simulink model "controller_v11_run"  (R2023a)
settings: Solver=ode4  StartTime=0.0  StopTime=5  FixedStep=0.00001  RelTol=1e-3
values from neighbouring files (symbols this model uses):
  m = 6    [coordinator_v2.m]
  N = 10    [coordinator_v2.m]
undefined symbols (not defined in the file or in its folder): PD_result, sd, X, Y, Z
libraries: sm_lib x191, nesl_utility x71
(part 1 of 5)
settings Model: Creator=25394  LastModifiedBy=shiyi
settings OptimizationCC: ReuseModelBlockBuffer=off

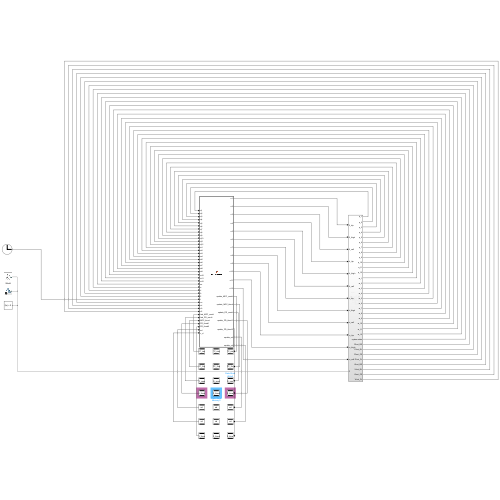
[thumbnail: Simulink's stored preview of the top-level diagram]
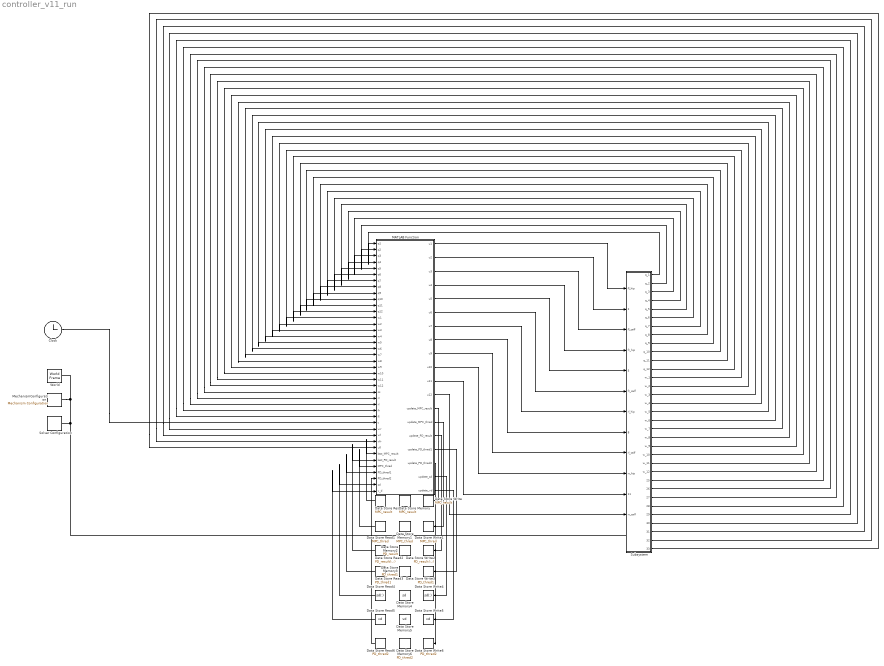
== system controller_v11_run ==
  Clock : Clock
  Data Store Memory : DataStoreMemory  DataStoreName=MPC_result  WriteAfterWriteMsg=warning  InitialValue=[0; 0; 0; 0; 0; 0; 0; 0; 0; 0; 0; 0]  ShowAdditionalParam=off
  Data Store Memory1 : DataStoreMemory  DataStoreName=MPC_thred  WriteAfterWriteMsg=warning  ShowAdditionalParam=off
  Data Store Memory2 : DataStoreMemory  DataStoreName=PD_result  WriteAfterWriteMsg=warning  InitialValue=zeros(24,14)  ShowAdditionalParam=off
  Data Store Memory3 : DataStoreMemory  DataStoreName=PD_thred1  WriteAfterWriteMsg=warning  ShowAdditionalParam=off
  Data Store Memory4 : DataStoreMemory  DataStoreName=sd  WriteAfterWriteMsg=warning  InitialValue=[0.1902; 0; 0.29; 0; 0; 0; 0; 0; 0; 0; 0; 0; 9.81]  ShowAdditionalParam=off
  Data Store Memory5 : DataStoreMemory  DataStoreName=vd  WriteAfterWriteMsg=warning  ShowAdditionalParam=off
  Data Store Memory6 : DataStoreMemory  DataStoreName=PD_thred2  WriteAfterWriteMsg=warning  ShowAdditionalParam=off
  Data Store Read : DataStoreRead  DataStoreName=MPC_result  IndexOptions=Index vector (dialog)  Indices=1  OutputSizes=1
  Data Store Read1 : DataStoreRead  DataStoreName=MPC_thred  IndexOptions=Index vector (dialog)  Indices=1  OutputSizes=1
  Data Store Read2 : DataStoreRead  DataStoreName=PD_result  DataStoreElements=PD_result(:,:)  IndexOptions=Index vector (dialog)  Indices=1  OutputSizes=1
  Data Store Read3 : DataStoreRead  DataStoreName=PD_thred1  IndexOptions=Index vector (dialog)  Indices=1  OutputSizes=1
  Data Store Read4 : DataStoreRead  DataStoreName=sd  DataStoreElements=sd(:)  IndexOptions=Index vector (dialog)  Indices=1  OutputSizes=1
  Data Store Read5 : DataStoreRead  DataStoreName=vd  DataStoreElements=vd  IndexOptions=Index vector (dialog)  Indices=1  OutputSizes=1
  Data Store Read6 : DataStoreRead  DataStoreName=PD_thred2  IndexOptions=Index vector (dialog)  Indices=1  OutputSizes=1
  Data Store Write : DataStoreWrite  DataStoreName=MPC_result  IndexOptions=Index vector (dialog)  Indices=1  OutputSizes=1
  Data Store Write1 : DataStoreWrite  DataStoreName=MPC_thred  IndexOptions=Index vector (dialog)  Indices=1  OutputSizes=1
  Data Store Write2 : DataStoreWrite  DataStoreName=PD_result  DataStoreElements=PD_result(:,:)  IndexOptions=Index vector (dialog)  Indices=1  OutputSizes=1
  Data Store Write3 : DataStoreWrite  DataStoreName=PD_thred1  IndexOptions=Index vector (dialog)  Indices=1  OutputSizes=1
  Data Store Write4 : DataStoreWrite  DataStoreName=sd  DataStoreElements=sd(:)  IndexOptions=Index vector (dialog)  Indices=1  OutputSizes=1
  Data Store Write5 : DataStoreWrite  DataStoreName=vd  DataStoreElements=vd  IndexOptions=Index vector (dialog)  Indices=1  OutputSizes=1
  Data Store Write6 : DataStoreWrite  DataStoreName=PD_thred2  IndexOptions=Index vector (dialog)  Indices=1  OutputSizes=1
  MATLAB Function : MATLAB Function  TreatAsAtomicUnit=on
  MechanismConfiguration : sm_lib/Utilities/Mechanism Configuration  UniformGravity=Constant  GravityVector=[0 0 -9.80665]  GravityVectorUnits=m/s^2  LinearizationDelta=0.001  JointModeTransitionNonlinearIterations=2
  Solver Configuration : nesl_utility/Solver Configuration  PhysicalDomain=network_engine_domain  SubClassName=solver  LeftPortType=input  RightPortType=generic  Tones=[]  Harmonics=[]  SimulateNoise=off  Profile=off  UseLocalSampling=off  EnableSwitchedLinearOptims=on  FrequencyDomain=off  UseCCode=off  RelTol=0.001  AbsTol=0.001  MinStep=1e-09  ToWorkspace=off  RevertToSquareIcSolve=off  NumHomotopyIterations=100  PhasorMode=off  PhasorModeNumHarmonics=1  ConsistencySolver=NEWTON_XTOL_AFTER_FTOL  IndexReductionMethod=DerivativeReplacement  DoDC=off  ResidualTolerance=1e-09  ConsistencyTolSource=GLOBAL  ConsistencyAbsTol=0.001  ConsistencyRelTol=0.001  ConsistencyTolFactor=0.001  UseLocalSolver=off  LocalSolverChoice=NE_BACKWARD_EULER_ADVANCER  ResolveIndetEquations=on  FunctionEvalNumThread=1  LocalSolverSampleTime=0.001  DoFixedCost=off  MaxNonlinIter=3  MaxModeIter=2  ComputeImpulses=off  ImpulseIterations=2  LinearAlgebra=auto  LinearAlgebraNumThread=0  EquationFormulation=NE_TIME_EF  DelaysMemoryBudget=1024  AutomaticFiltering=on  FilteringTimeConstant=0.001  PartitionStorageMethod=AS_NEEDED  PartitionMemoryBudget=1024  PartitionMethod=ROBUST
  Subsystem : Subsystem
  World : sm_lib/Frames and Transforms/World Frame
  wires:
  Clock/1 -> MATLAB Function/30(t)
  MATLAB Function/1(u1) -> Subsystem/1(fl_hip)
  MATLAB Function/2(u2) -> Subsystem/2(fl_thigh)
  MATLAB Function/3(u3) -> Subsystem/3(fl_calf)
  MATLAB Function/4(u4) -> Subsystem/4(fr_hip)
  MATLAB Function/5(u5) -> Subsystem/5(fr_thigh)
  MATLAB Function/6(u6) -> Subsystem/6(fr_calf)
  MATLAB Function/7(u7) -> Subsystem/7(rl_hip)
  MATLAB Function/8(u8) -> Subsystem/8(rl_thigh)
  MATLAB Function/9(u9) -> Subsystem/9(rl_calf)
  MATLAB Function/10(u10) -> Subsystem/10(rr_hip)
  MATLAB Function/11(u11) -> Subsystem/11(rr_thigh)
  MATLAB Function/12(u12) -> Subsystem/12(rr_calf)
  Subsystem/1(q_1) -> MATLAB Function/1(q1)
  Subsystem/2(q_2) -> MATLAB Function/2(q2)
  Subsystem/3(q_3) -> MATLAB Function/3(q3)
  Subsystem/4(q_4) -> MATLAB Function/4(q4)
  Subsystem/5(q_5) -> MATLAB Function/5(q5)
  Subsystem/6(q_6) -> MATLAB Function/6(q6)
  Subsystem/7(q_7) -> MATLAB Function/7(q7)
  Subsystem/8(q_8) -> MATLAB Function/8(q8)
  Subsystem/9(q_9) -> MATLAB Function/9(q9)
  Subsystem/10(q_10) -> MATLAB Function/10(q10)
  Subsystem/11(q_11) -> MATLAB Function/11(q11)
  Subsystem/12(q_12) -> MATLAB Function/12(q12)
  Subsystem/13(w_1) -> MATLAB Function/13(w1)
  Subsystem/14(w_2) -> MATLAB Function/14(w2)
  Subsystem/15(w_3) -> MATLAB Function/15(w3)
  Subsystem/16(w_4) -> MATLAB Function/16(w4)
  Subsystem/17(w_5) -> MATLAB Function/17(w5)
  Subsystem/18(w_6) -> MATLAB Function/18(w6)
  Subsystem/19(w_7) -> MATLAB Function/19(w7)
  Subsystem/20(w_8) -> MATLAB Function/20(w8)
  Subsystem/21(w_9) -> MATLAB Function/21(w9)
  Subsystem/22(w_10) -> MATLAB Function/22(w10)
  Subsystem/23(w_11) -> MATLAB Function/23(w11)
  Subsystem/24(w_12) -> MATLAB Function/24(w12)
  Subsystem/25(system state) -> MATLAB Function/25(ss)
  Subsystem/26(Pfoot_RR) -> MATLAB Function/26(rr)
  Subsystem/27(Pfoot_RL) -> MATLAB Function/27(rl)
  Subsystem/28(Pfoot_FR) -> MATLAB Function/28(fr)
  Subsystem/29(Pfoot_FL) -> MATLAB Function/29(fl)
  Subsystem/30(Vfoot_RR) -> MATLAB Function/31(vrr)
  Subsystem/31(Vfoot_RL) -> MATLAB Function/32(vrl)
  Subsystem/32(Vfoot_FR) -> MATLAB Function/33(vfr)
  Subsystem/33(Vfoot_FL) -> MATLAB Function/34(vfl)
  MATLAB Function/13(update_MPC_result) -> Data Store Write/1
  Data Store Read/1 -> MATLAB Function/35(last_MPC_result)
  Data Store Read1/1 -> MATLAB Function/37(MPC_thred)
  MATLAB Function/14(update_MPC_thred) -> Data Store Write1/1
  MATLAB Function/15(update_PD_result) -> Data Store Write2/1
  Data Store Read2/1 -> MATLAB Function/36(last_PD_result)
  MATLAB Function/16(update_PD_thred1) -> Data Store Write3/1
  Data Store Read3/1 -> MATLAB Function/38(PD_thred1)
  MATLAB Function/18(update_sd) -> Data Store Write4/1
  Data Store Read4/1 -> MATLAB Function/40(sd)
  MATLAB Function/19(update_vd) -> Data Store Write5/1
  Data Store Read5/1 -> MATLAB Function/41(v_d)
  MATLAB Function/17(update_PD_thred2) -> Data Store Write6/1
  Data Store Read6/1 -> MATLAB Function/39(PD_thred2)
  connections:
  World/RConn1 -- Subsystem/LConn1 -- Solver Configuration/RConn1 -- MechanismConfiguration/RConn1
